simulink model "regulator_LQR"  (Simulink 10.0)
settings: Solver=ode45  StartTime=0.0  StopTime=tsim  RelTol=1e-3  EnableMultiTasking=on
values from neighbouring files (symbols this model uses):
  C_states = eye(2)    [es2.m]
  D_states = [0 0]'    [es2.m]
  Klqr1 = lqr(A,B,Q,R)    [es2.m]
  sat_max = inf    [es2.m]
  sat_min = -inf    [es2.m]
  x0 = [0 10]    [es2.m]
undefined symbols (not defined in the file or in its folder): A, B, C
settings Model: Creator=Administrator  LastModifiedBy=Chiara
settings DataIOCC: LimitDataPoints=on  SignalLoggingSaveFormat=ModelDataLogs
settings OptimizationCC: ExpressionDepthLimit=2147483647  InitFltsAndDblsToZero=on
settings DebuggingCC: SolverPrmCheckMsg=warning  FcnCallInpInsideContextMsg=warning  StateNameClashWarn=warning
settings GRTTargetCC: GeneratePreprocessorConditionals=Disable all
settings ConfigComp: CovExternalEMLEnable=off  CovSFcnEnable=off

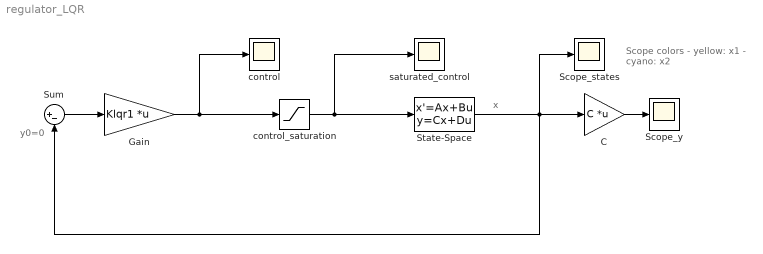
== system regulator_LQR ==
  note: y0=0
  note: x
  note: Scope colors
      | - yellow: x1
      | - cyano: x2
  C : Gain  Gain=C  Multiplication=Matrix(K*u)
  Gain : Gain  Gain=Klqr1  Multiplication=Matrix(K*u)
  Scope_states : Scope
  Scope_y : Scope
  "State-Space " : StateSpace  A=A  B=B  C=C_states  D=D_states  InitialCondition=x0
  Sum : Sum  Inputs=|+-
  control : Scope
  control_saturation : Saturate  UpperLimit=sat_max  LowerLimit=sat_min
  saturated_control : Scope
  wires:
  control_saturation/1 -> "State-Space "/1, saturated_control/1
  Gain/1 -> control_saturation/1, control/1
  Sum/1 -> Gain/1
  "State-Space "/1 -> Scope_states/1, C/1, Sum/2
  C/1 -> Scope_y/1
